simulink model "electricUAV"  (R2019a)
settings: Solver=VariableStepAuto  StartTime=0.0  StopTime=10.0  RelTol=1e-3
model workspace (MAT data in the model file):
  Var = 0
  architecture_gsCommands = Simulink.Bus
  architecture_gsCommands.Alignment = -1
  architecture_gsCommands.Elements_internal(1) = Simulink.BusElement
  architecture_gsCommands.Elements_internal(1).DimensionsMode = 'Fixed'
  architecture_gsCommands.Elements_internal(1).SamplingMode = 'Sample based'
  architecture_gsCommands.Elements_internal(1).SampleTime = -1
  architecture_gsCommands.Elements_internal(1).Name = 'apConfigParams'
  architecture_gsCommands.Elements_internal(1).DataType_internal = 'Bus: param_value_bus'
  architecture_gsCommands.Elements_internal(1).Complexity = 'real'
  architecture_gsCommands.Elements_internal(1).Dimensions = 1
  architecture_gsCommands.Elements_internal(2) = Simulink.BusElement
  architecture_gsCommands.Elements_internal(2).DimensionsMode = 'Fixed'
  architecture_gsCommands.Elements_internal(2).SamplingMode = 'Sample based'
  architecture_gsCommands.Elements_internal(2).SampleTime = -1
  architecture_gsCommands.Elements_internal(2).Name = 'gsCommands'
  architecture_gsCommands.Elements_internal(2).DataType_internal = 'Bus: gs_commands_bus'
  architecture_gsCommands.Elements_internal(2).Complexity = 'real'
  architecture_gsCommands.Elements_internal(2).Dimensions = 1
  architecture_gsCommands.Elements_internal(3) = Simulink.BusElement
  architecture_gsCommands.Elements_internal(3).DimensionsMode = 'Fixed'
  architecture_gsCommands.Elements_internal(3).SamplingMode = 'Sample based'
  architecture_gsCommands.Elements_internal(3).SampleTime = -1
  architecture_gsCommands.Elements_internal(3).Name = 'uavMission'
  architecture_gsCommands.Elements_internal(3).DataType_internal = 'Bus: mission_item_bus'
  architecture_gsCommands.Elements_internal(3).Complexity = 'real'
  architecture_gsCommands.Elements_internal(3).Dimensions = 1
  architecture_gsCommands.DataScope = 'Auto'
  ctrlSrfcDeflection = Simulink.Bus
  ctrlSrfcDeflection.Alignment = -1
  ctrlSrfcDeflection.Elements_internal(1) = Simulink.BusElement
  ctrlSrfcDeflection.Elements_internal(1).DimensionsMode = 'Fixed'
  ctrlSrfcDeflection.Elements_internal(1).SamplingMode = 'Sample based'
  ctrlSrfcDeflection.Elements_internal(1).SampleTime = -1
  ctrlSrfcDeflection.Elements_internal(1).Name = 'dA_dF'
  ctrlSrfcDeflection.Elements_internal(1).DataType_internal = 'double'
  ctrlSrfcDeflection.Elements_internal(1).Complexity = 'real'
  ctrlSrfcDeflection.Elements_internal(1).Dimensions = 1
  ctrlSrfcDeflection.Elements_internal(2) = Simulink.BusElement
  ctrlSrfcDeflection.Elements_internal(2).DimensionsMode = 'Fixed'
  ctrlSrfcDeflection.Elements_internal(2).SamplingMode = 'Sample based'
  ctrlSrfcDeflection.Elements_internal(2).SampleTime = -1
  ctrlSrfcDeflection.Elements_internal(2).Name = 'dT'
  ctrlSrfcDeflection.Elements_internal(2).DataType_internal = 'double'
  ctrlSrfcDeflection.Elements_internal(2).Complexity = 'real'
  ctrlSrfcDeflection.Elements_internal(2).Dimensions = 1
  ctrlSrfcDeflection.Elements_internal(3) = Simulink.BusElement
  ctrlSrfcDeflection.Elements_internal(3).DimensionsMode = 'Fixed'
  ctrlSrfcDeflection.Elements_internal(3).SamplingMode = 'Sample based'
  ctrlSrfcDeflection.Elements_internal(3).SampleTime = -1
  ctrlSrfcDeflection.Elements_internal(3).Name = 'dR_dE'
  ctrlSrfcDeflection.Elements_internal(3).DataType_internal = 'double'
  ctrlSrfcDeflection.Elements_internal(3).Complexity = 'real'
  ctrlSrfcDeflection.Elements_internal(3).Dimensions = 1
  ctrlSrfcDeflection.DataScope = 'Auto'
  gs_commands_bus = Simulink.Bus
  gs_commands_bus.Alignment = -1
  gs_commands_bus.Elements_internal(1) = Simulink.BusElement
  gs_commands_bus.Elements_internal(1).DimensionsMode = 'Fixed'
  gs_commands_bus.Elements_internal(1).SamplingMode = 'Sample based'
  gs_commands_bus.Elements_internal(1).SampleTime = -1
  gs_commands_bus.Elements_internal(1).Description = 'Return to Base Command'
  gs_commands_bus.Elements_internal(1).Name = 'RTB'
  gs_commands_bus.Elements_internal(1).DataType_internal = 'uint8'
  gs_commands_bus.Elements_internal(1).Complexity = 'real'
  gs_commands_bus.Elements_internal(1).Dimensions = 1
  gs_commands_bus.Elements_internal(2) = Simulink.BusElement
  gs_commands_bus.Elements_internal(2).DimensionsMode = 'Fixed'
  gs_commands_bus.Elements_internal(2).SamplingMode = 'Sample based'
  gs_commands_bus.Elements_internal(2).SampleTime = -1
  gs_commands_bus.Elements_internal(2).Description = 'Airspeed Commanded by the GS'
  gs_commands_bus.Elements_internal(2).Name = 'U_c'
  gs_commands_bus.Elements_internal(2).DataType_internal = 'single'
  gs_commands_bus.Elements_internal(2).Complexity = 'real'
  gs_commands_bus.Elements_internal(2).Dimensions = 1
  gs_commands_bus.Elements_internal(3) = Simulink.BusElement
  gs_commands_bus.Elements_internal(3).DimensionsMode = 'Fixed'
  gs_commands_bus.Elements_internal(3).SamplingMode = 'Sample based'
  gs_commands_bus.Elements_internal(3).SampleTime = -1
  gs_commands_bus.Elements_internal(3).Description = 'Turnrate command when in mid Level Commands guidance mode'
  gs_commands_bus.Elements_internal(3).Name = 'psiDot_c_mdiLevel'
  gs_commands_bus.Elements_internal(3).DataType_internal = 'single'
  gs_commands_bus.Elements_internal(3).Complexity = 'real'
  gs_commands_bus.Elements_internal(3).Dimensions = 1
  gs_commands_bus.Elements_internal(4) = Simulink.BusElement
  gs_commands_bus.Elements_internal(4).DimensionsMode = 'Fixed'
  gs_commands_bus.Elements_internal(4).SamplingMode = 'Sample based'
  gs_commands_bus.Elements_internal(4).SampleTime = -1
  gs_commands_bus.Elements_internal(4).Description = 'Commanded altitude when in Mid Level Commands Mode. Also used as the altitude for RTB'
  gs_commands_bus.Elements_internal(4).Name = 'h_c_midLevel'
  gs_commands_bus.Elements_internal(4).DataType_internal = 'single'
  gs_commands_bus.Elements_internal(4).Complexity = 'real'
  gs_commands_bus.Elements_internal(4).Dimensions = 1
  gs_commands_bus.Elements_internal(5) = Simulink.BusElement
  gs_commands_bus.Elements_internal(5).DimensionsMode = 'Fixed'
  gs_commands_bus.Elements_internal(5).SamplingMode = 'Sample based'
  gs_commands_bus.Elements_internal(5).SampleTime = -1
  gs_commands_bus.Elements_internal(5).Name = 'isManualModeOn'
  gs_commands_bus.Elements_internal(5).DataType_internal = 'uint8'
  gs_commands_bus.Elements_internal(5).Complexity = 'real'
  gs_commands_bus.Elements_internal(5).Dimensions = 1
  gs_commands_bus.Elements_internal(6) = Simulink.BusElement
  gs_commands_bus.Elements_internal(6).DimensionsMode = 'Fixed'
  gs_commands_bus.Elements_internal(6).SamplingMode = 'Sample based'
  gs_commands_bus.Elements_internal(6).SampleTime = -1
  gs_commands_bus.Elements_internal(6).Name = 'viewPointIdx'
  gs_commands_bus.Elements_internal(6).DataType_internal = 'uint8'
  gs_commands_bus.Elements_internal(6).Complexity = 'real'
  gs_commands_bus.Elements_internal(6).Dimensions = 1
  gs_commands_bus.Elements_internal(7) = Simulink.BusElement
  gs_commands_bus.Elements_internal(7).DimensionsMode = 'Fixed'
  gs_commands_bus.Elements_internal(7).SamplingMode = 'Sample based'
  gs_commands_bus.Elements_internal(7).SampleTime = -1
  gs_commands_bus.Elements_internal(7).Name = 'guidanceMode'
  gs_commands_bus.Elements_internal(7).DataType_internal = 'uint8'
  gs_commands_bus.Elements_internal(7).Complexity = 'real'
  gs_commands_bus.Elements_internal(7).Dimensions = 1
  gs_commands_bus.DataScope = 'Auto'
  lightCmds = Simulink.Bus
  lightCmds.Alignment = -1
  lightCmds.Elements_internal(1) = Simulink.BusElement
  lightCmds.Elements_internal(1).DimensionsMode = 'Fixed'
  lightCmds.Elements_internal(1).SamplingMode = 'Sample based'
  lightCmds.Elements_internal(1).SampleTime = -1
  lightCmds.Elements_internal(1).Name = 'NavigationLights'
  lightCmds.Elements_internal(1).DataType_internal = 'double'
  lightCmds.Elements_internal(1).Complexity = 'real'
  lightCmds.Elements_internal(1).Dimensions = 1
  lightCmds.Elements_internal(2) = Simulink.BusElement
  lightCmds.Elements_internal(2).DimensionsMode = 'Fixed'
  lightCmds.Elements_internal(2).SamplingMode = 'Sample based'
  lightCmds.Elements_internal(2).SampleTime = -1
  lightCmds.Elements_internal(2).Name = 'LandingStrobe'
  lightCmds.Elements_internal(2).DataType_internal = 'double'
  lightCmds.Elements_internal(2).Complexity = 'real'
  lightCmds.Elements_internal(2).Dimensions = 1
  lightCmds.DataScope = 'Auto'
  mission_item_bus = Simulink.Bus
  mission_item_bus.Alignment = -1
  mission_item_bus.Elements_internal(1) = Simulink.BusElement
  mission_item_bus.Elements_internal(1).DimensionsMode = 'Fixed'
  mission_item_bus.Elements_internal(1).SamplingMode = 'Sample based'
  mission_item_bus.Elements_internal(1).SampleTime = -1
  mission_item_bus.Elements_internal(1).Description = 'PARAM1, see MAV_CMD enum'
  mission_item_bus.Elements_internal(1).Name = 'param1'
  mission_item_bus.Elements_internal(1).DataType_internal = 'single'
  mission_item_bus.Elements_internal(1).Complexity = 'real'
  mission_item_bus.Elements_internal(1).Dimensions = 1
  mission_item_bus.Elements_internal(2) = Simulink.BusElement
  mission_item_bus.Elements_internal(2).DimensionsMode = 'Fixed'
  mission_item_bus.Elements_internal(2).SamplingMode = 'Sample based'
  mission_item_bus.Elements_internal(2).SampleTime = -1
  mission_item_bus.Elements_internal(2).Description = 'PARAM4, see MAV_CMD enum'
  mission_item_bus.Elements_internal(2).Name = 'param4'
  mission_item_bus.Elements_internal(2).DataType_internal = 'single'
  mission_item_bus.Elements_internal(2).Complexity = 'real'
  mission_item_bus.Elements_internal(2).Dimensions = 1
  mission_item_bus.Elements_internal(3) = Simulink.BusElement
  mission_item_bus.Elements_internal(3).DimensionsMode = 'Fixed'
  mission_item_bus.Elements_internal(3).SamplingMode = 'Sample based'
  mission_item_bus.Elements_internal(3).SampleTime = -1
  mission_item_bus.Elements_internal(3).Description = 'PARAM3, see MAV_CMD enum'
  mission_item_bus.Elements_internal(3).Name = 'param3'
  mission_item_bus.Elements_internal(3).DataType_internal = 'single'
  mission_item_bus.Elements_internal(3).Complexity = 'real'
  mission_item_bus.Elements_internal(3).Dimensions = 1
  mission_item_bus.Elements_internal(4) = Simulink.BusElement
  mission_item_bus.Elements_internal(4).DimensionsMode = 'Fixed'
  mission_item_bus.Elements_internal(4).SamplingMode = 'Sample based'
  mission_item_bus.Elements_internal(4).SampleTime = -1
  mission_item_bus.Elements_internal(4).Description = 'false:0, true:1'
  mission_item_bus.Elements_internal(4).Name = 'current'
  mission_item_bus.Elements_internal(4).DataType_internal = 'uint8'
  mission_item_bus.Elements_internal(4).Complexity = 'real'
  mission_item_bus.Elements_internal(4).Dimensions = 1
  mission_item_bus.Elements_internal(5) = Simulink.BusElement
  mission_item_bus.Elements_internal(5).DimensionsMode = 'Fixed'
  mission_item_bus.Elements_internal(5).SamplingMode = 'Sample based'
  mission_item_bus.Elements_internal(5).SampleTime = -1
  mission_item_bus.Elements_internal(5).Description = 'PARAM2, see MAV_CMD enum'
  mission_item_bus.Elements_internal(5).Name = 'param2'
  mission_item_bus.Elements_internal(5).DataType_internal = 'single'
  mission_item_bus.Elements_internal(5).Complexity = 'real'
  mission_item_bus.Elements_internal(5).Dimensions = 1
  mission_item_bus.Elements_internal(6) = Simulink.BusElement
  mission_item_bus.Elements_internal(6).DimensionsMode = 'Fixed'
  mission_item_bus.Elements_internal(6).SamplingMode = 'Sample based'
  mission_item_bus.Elements_internal(6).SampleTime = -1
  mission_item_bus.Elements_internal(6).Description = 'PARAM5 / local: x position, global: latitude'
  mission_item_bus.Elements_internal(6).Name = 'x'
  mission_item_bus.Elements_internal(6).DataType_internal = 'single'
  mission_item_bus.Elements_internal(6).Complexity = 'real'
  mission_item_bus.Elements_internal(6).Dimensions = 1
  mission_item_bus.Elements_internal(7) = Simulink.BusElement
  mission_item_bus.Elements_internal(7).DimensionsMode = 'Fixed'
  mission_item_bus.Elements_internal(7).SamplingMode = 'Sample based'
  mission_item_bus.Elements_internal(7).SampleTime = -1
  mission_item_bus.Elements_internal(7).Description = 'PARAM6 / y position: global: longitude'
  mission_item_bus.Elements_internal(7).Name = 'y'
  mission_item_bus.Elements_internal(7).DataType_internal = 'single'
  mission_item_bus.Elements_internal(7).Complexity = 'real'
  mission_item_bus.Elements_internal(7).Dimensions = 1
  mission_item_bus.Elements_internal(8) = Simulink.BusElement
  mission_item_bus.Elements_internal(8).DimensionsMode = 'Fixed'
  mission_item_bus.Elements_internal(8).SamplingMode = 'Sample based'
  mission_item_bus.Elements_internal(8).SampleTime = -1
  mission_item_bus.Elements_internal(8).Description = 'The scheduled action for the waypoint. see MAV_CMD in common.xml MAVLink specs'
  mission_item_bus.Elements_internal(8).Name = 'command'
  mission_item_bus.Elements_internal(8).DataType_internal = 'uint16'
  mission_item_bus.Elements_internal(8).Complexity = 'real'
  mission_item_bus.Elements_internal(8).Dimensions = 1
  mission_item_bus.Elements_internal(9) = Simulink.BusElement
  mission_item_bus.Elements_internal(9).DimensionsMode = 'Fixed'
  mission_item_bus.Elements_internal(9).SamplingMode = 'Sample based'
  mission_item_bus.Elements_internal(9).SampleTime = -1
  mission_item_bus.Elements_internal(9).Description = 'PARAM7 / z position: global: altitude (relative or absolute, depending on frame.'
  mission_item_bus.Elements_internal(9).Name = 'z'
  mission_item_bus.Elements_internal(9).DataType_internal = 'single'
  mission_item_bus.Elements_internal(9).Complexity = 'real'
  mission_item_bus.Elements_internal(9).Dimensions = 1
  mission_item_bus.Elements_internal(10) = Simulink.BusElement
  mission_item_bus.Elements_internal(10).DimensionsMode = 'Fixed'
  mission_item_bus.Elements_internal(10).SamplingMode = 'Sample based'
  mission_item_bus.Elements_internal(10).SampleTime = -1
  mission_item_bus.Elements_internal(10).Description = 'System ID'
  mission_item_bus.Elements_internal(10).Name = 'target_system'
  mission_item_bus.Elements_internal(10).DataType_internal = 'uint8'
  mission_item_bus.Elements_internal(10).Complexity = 'real'
  mission_item_bus.Elements_internal(10).Dimensions = 1
  mission_item_bus.Elements_internal(11) = Simulink.BusElement
  mission_item_bus.Elements_internal(11).DimensionsMode = 'Fixed'
  mission_item_bus.Elements_internal(11).SamplingMode = 'Sample based'
  mission_item_bus.Elements_internal(11).SampleTime = -1
  mission_item_bus.Elements_internal(11).Description = 'Sequence'
  mission_item_bus.Elements_internal(11).Name = 'seq'
  mission_item_bus.Elements_internal(11).DataType_internal = 'uint16'
  mission_item_bus.Elements_internal(11).Complexity = 'real'
  mission_item_bus.Elements_internal(11).Dimensions = 1
  mission_item_bus.Elements_internal(12) = Simulink.BusElement
  mission_item_bus.Elements_internal(12).DimensionsMode = 'Fixed'
  mission_item_bus.Elements_internal(12).SamplingMode = 'Sample based'
  mission_item_bus.Elements_internal(12).SampleTime = -1
  mission_item_bus.Elements_internal(12).Description = 'Mission type, see MAV_MISSION_TYPE'
  mission_item_bus.Elements_internal(12).Name = 'mission_type'
  mission_item_bus.Elements_internal(12).DataType_internal = 'uint8'
  mission_item_bus.Elements_internal(12).Complexity = 'real'
  mission_item_bus.Elements_internal(12).Dimensions = 1
  mission_item_bus.Elements_internal(13) = Simulink.BusElement
  mission_item_bus.Elements_internal(13).DimensionsMode = 'Fixed'
  mission_item_bus.Elements_internal(13).SamplingMode = 'Sample based'
  mission_item_bus.Elements_internal(13).SampleTime = -1
  mission_item_bus.Elements_internal(13).Description = 'The coordinate system of the waypoint. see MAV_FRAME in mavlink_types.h'
  mission_item_bus.Elements_internal(13).Name = 'frame'
  mission_item_bus.Elements_internal(13).DataType_internal = 'uint8'
  mission_item_bus.Elements_internal(13).Complexity = 'real'
  mission_item_bus.Elements_internal(13).Dimensions = 1
  mission_item_bus.Elements_internal(14) = Simulink.BusElement
  mission_item_bus.Elements_internal(14).DimensionsMode = 'Fixed'
  mission_item_bus.Elements_internal(14).SamplingMode = 'Sample based'
  mission_item_bus.Elements_internal(14).SampleTime = -1
  mission_item_bus.Elements_internal(14).Description = 'Component ID'
  mission_item_bus.Elements_internal(14).Name = 'target_component'
  mission_item_bus.Elements_internal(14).DataType_internal = 'uint8'
  mission_item_bus.Elements_internal(14).Complexity = 'real'
  mission_item_bus.Elements_internal(14).Dimensions = 1
  mission_item_bus.Elements_internal(15) = Simulink.BusElement
  mission_item_bus.Elements_internal(15).DimensionsMode = 'Fixed'
  mission_item_bus.Elements_internal(15).SamplingMode = 'Sample based'
  mission_item_bus.Elements_internal(15).SampleTime = -1
  mission_item_bus.Elements_internal(15).Description = 'autocontinue to next wp'
  mission_item_bus.Elements_internal(15).Name = 'autocontinue'
  mission_item_bus.Elements_internal(15).DataType_internal = 'uint8'
  mission_item_bus.Elements_internal(15).Complexity = 'real'
  mission_item_bus.Elements_internal(15).Dimensions = 1
  mission_item_bus.DataScope = 'Auto'
  operatorCmds = Simulink.Bus
  operatorCmds.Alignment = -1
  operatorCmds.Elements_internal(1) = Simulink.BusElement
  operatorCmds.Elements_internal(1).DimensionsMode = 'Fixed'
  operatorCmds.Elements_internal(1).SamplingMode = 'Sample based'
  operatorCmds.Elements_internal(1).SampleTime = -1
  operatorCmds.Elements_internal(1).Name = 'RetractorCmds'
  operatorCmds.Elements_internal(1).DataType_internal = 'double'
  operatorCmds.Elements_internal(1).Complexity = 'real'
  operatorCmds.Elements_internal(1).Dimensions = 1
  operatorCmds.Elements_internal(2) = Simulink.BusElement
  operatorCmds.Elements_internal(2).DimensionsMode = 'Fixed'
  operatorCmds.Elements_internal(2).SamplingMode = 'Sample based'
  operatorCmds.Elements_internal(2).SampleTime = -1
  operatorCmds.Elements_internal(2).Name = 'PTZCmds'
  operatorCmds.Elements_internal(2).DataType_internal = 'double'
  operatorCmds.Elements_internal(2).Complexity = 'real'
  operatorCmds.Elements_internal(2).Dimensions = 1
  operatorCmds.DataScope = 'Auto'
  param_value_bus = Simulink.Bus
  param_value_bus.Alignment = -1
  param_value_bus.Elements_internal(1) = Simulink.BusElement
  param_value_bus.Elements_internal(1).DimensionsMode = 'Fixed'
  param_value_bus.Elements_internal(1).SamplingMode = 'Sample based'
  param_value_bus.Elements_internal(1).SampleTime = -1
  param_value_bus.Elements_internal(1).Description = 'Onboard parameter value'
  param_value_bus.Elements_internal(1).Name = 'param_value'
  param_value_bus.Elements_internal(1).DataType_internal = 'single'
  param_value_bus.Elements_internal(1).Complexity = 'real'
  param_value_bus.Elements_internal(1).Dimensions = 1
  param_value_bus.Elements_internal(2) = Simulink.BusElement
  param_value_bus.Elements_internal(2).DimensionsMode = 'Fixed'
  param_value_bus.Elements_internal(2).SamplingMode = 'Sample based'
  param_value_bus.Elements_internal(2).SampleTime = -1
  param_value_bus.Elements_internal(2).Description = 'Index of this onboard parameter'
  param_value_bus.Elements_internal(2).Name = 'param_index'
  param_value_bus.Elements_internal(2).DataType_internal = 'uint16'
  param_value_bus.Elements_internal(2).Complexity = 'real'
  param_value_bus.Elements_internal(2).Dimensions = 1
  param_value_bus.Elements_internal(3) = Simulink.BusElement
  param_value_bus.Elements_internal(3).DimensionsMode = 'Fixed'
  param_value_bus.Elements_internal(3).SamplingMode = 'Sample based'
  param_value_bus.Elements_internal(3).SampleTime = -1
  param_value_bus.Elements_internal(3).Description = 'Total number of onboard parameters'
  param_value_bus.Elements_internal(3).Name = 'param_count'
  param_value_bus.Elements_internal(3).DataType_internal = 'uint16'
  param_value_bus.Elements_internal(3).Complexity = 'real'
  param_value_bus.Elements_internal(3).Dimensions = 1
  param_value_bus.Elements_internal(4) = Simulink.BusElement
  param_value_bus.Elements_internal(4).DimensionsMode = 'Fixed'
  param_value_bus.Elements_internal(4).SamplingMode = 'Sample based'
  param_value_bus.Elements_internal(4).SampleTime = -1
  param_value_bus.Elements_internal(4).Description = 'Onboard parameter id, terminated by NULL if the length is less than 16 human-readable chars and WITHOUT null termination (NULL) byte if the length is exactly 16 chars - applications have to provide 16+1 bytes storage if the ID is stored as string'
  param_value_bus.Elements_internal(4).Name = 'param_id'
  param_value_bus.Elements_internal(4).DataType_internal = 'int8'
  param_value_bus.Elements_internal(4).Complexity = 'real'
  param_value_bus.Elements_internal(4).Dimensions = 16
  param_value_bus.Elements_internal(5) = Simulink.BusElement
  param_value_bus.Elements_internal(5).DimensionsMode = 'Fixed'
  param_value_bus.Elements_internal(5).SamplingMode = 'Sample based'
  param_value_bus.Elements_internal(5).SampleTime = -1
  param_value_bus.Elements_internal(5).Description = 'Onboard parameter type: see the MAV_PARAM_TYPE enum for supported data types.'
  param_value_bus.Elements_internal(5).Name = 'param_type'
  param_value_bus.Elements_internal(5).DataType_internal = 'uint8'
  param_value_bus.Elements_internal(5).Complexity = 'real'
  param_value_bus.Elements_internal(5).Dimensions = 1
  param_value_bus.DataScope = 'Auto'
settings Model: OrderedModelArguments=off  Creator=pshukla  LastModifiedBy=lizarraga

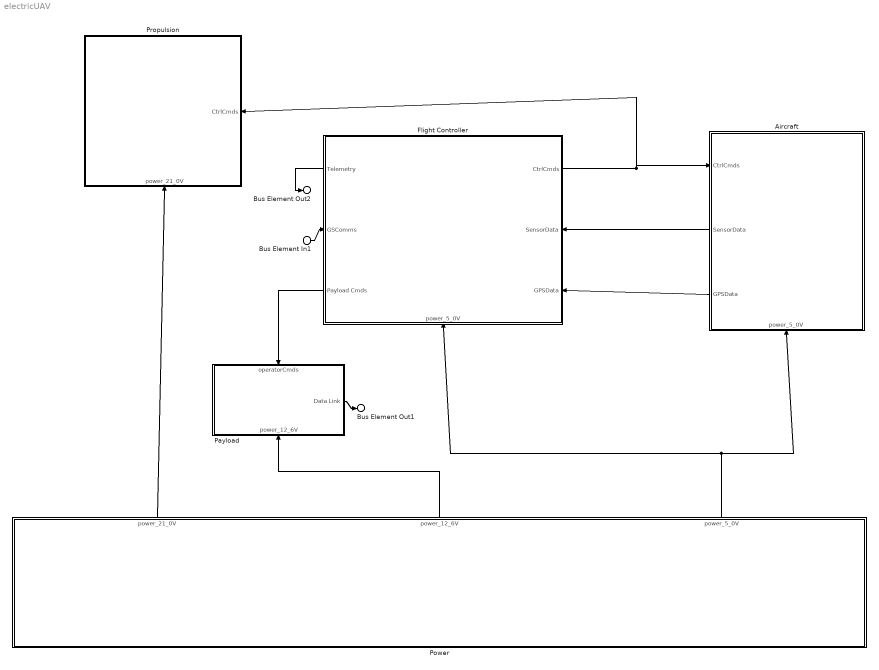
== system electricUAV ==
  Bus Element In1 : Inport  PortName=GS Communication
  Aircraft : Subsystem
      settings: PortSchema="{\"entries\":[{\"content\":{\"headerSize\":26,\"margin\":15,\"minimumSpacing\":25,\"sides\":[{\"content\":{\"connectorIds\":[\"In2\",\"Out1\",\"Out2\"]},\"type\":\"ConnectorPlacement.EquallySpacedRectSide\",\"uuid\":\"5864bfaa-27bf-4dc4-ac35-2a67754e9235\"},{\"content\":{\"connectorIds\":[],\"side\":\"RIGHT\"},\"type\":\"ConnectorPlacement.EquallySpacedRectSide\",\"uuid\":\"1b67a812-6201-4dd3-b7dd-96f38505ac3f\"},{\"content\":{\"connectorIds\":[],\"side\":\"TOP\"},\"type\":\"ConnectorPlacement.EquallySpacedRectSide\",\"uuid\":\"0ccb1f06-40bd-43a7-ae7f-56a6fcc507bd\"},{\"content\":{\"connectorIds\":[\"In1\"],\"side\":\"BOTTOM\"},\"type\":\"ConnectorPlacement.EquallySpacedRectSide\",\"uuid\":\"b85c3588-b067-49c6-8cfc-8b359955ba08\"}]},\"type\":\"ConnectorPlacement.EquallySpacedConnector\",\"uuid\":\"adb7d5a4-9c70-4105-bc6e-780ed1523c48\"}],\"packageUris\":[\"http:\\/\\/schema.mathworks.com\\/mf0\\/Connector\\/19700101\"],\"version\":\"1.0\"}"
  Flight Controller : Subsystem
      settings: PortSchema="{\"entries\":[{\"content\":{\"headerSize\":26,\"margin\":15,\"minimumSpacing\":25,\"sides\":[{\"content\":{\"connectorIds\":[\"Out3\",\"In4\",\"Out2\"]},\"type\":\"ConnectorPlacement.EquallySpacedRectSide\",\"uuid\":\"288187f8-f80a-4535-8eff-6998f4e932c0\"},{\"content\":{\"connectorIds\":[\"Out1\",\"In2\",\"In3\"],\"side\":\"RIGHT\"},\"type\":\"ConnectorPlacement.EquallySpacedRectSide\",\"uuid\":\"d1e22774-cdd2-4e71-94b1-3e938d9d16f6\"},{\"content\":{\"connectorIds\":[],\"side\":\"TOP\"},\"type\":\"ConnectorPlacement.EquallySpacedRectSide\",\"uuid\":\"890411bd-a9cd-40b1-a683-0574f0cd14d7\"},{\"content\":{\"connectorIds\":[\"In1\"],\"side\":\"BOTTOM\"},\"type\":\"ConnectorPlacement.EquallySpacedRectSide\",\"uuid\":\"5b2b87a3-00cb-493f-9187-a9231b1dbd9e\"}]},\"type\":\"ConnectorPlacement.EquallySpacedConnector\",\"uuid\":\"f677e6f7-ddb0-43ad-ab3a-7892dac74d79\"}],\"packageUris\":[\"http:\\/\\/schema.mathworks.com\\/mf0\\/Connector\\/19700101\"],\"version\":\"1.0\"}"
  Payload : Subsystem
      settings: PortSchema="{\"entries\":[{\"content\":{\"headerSize\":26,\"margin\":15,\"minimumSpacing\":25,\"sides\":[{\"content\":{\"connectorIds\":[]},\"type\":\"ConnectorPlacement.EquallySpacedRectSide\",\"uuid\":\"288187f8-f80a-4535-8eff-6998f4e932c0\"},{\"content\":{\"connectorIds\":[\"Out1\"],\"side\":\"RIGHT\"},\"type\":\"ConnectorPlacement.EquallySpacedRectSide\",\"uuid\":\"d1e22774-cdd2-4e71-94b1-3e938d9d16f6\"},{\"content\":{\"connectorIds\":[\"In2\"],\"side\":\"TOP\"},\"type\":\"ConnectorPlacement.EquallySpacedRectSide\",\"uuid\":\"890411bd-a9cd-40b1-a683-0574f0cd14d7\"},{\"content\":{\"connectorIds\":[\"In1\"],\"side\":\"BOTTOM\"},\"type\":\"ConnectorPlacement.EquallySpacedRectSide\",\"uuid\":\"ac2f29b9-61c6-4e35-85f4-3f1356623504\"}]},\"type\":\"ConnectorPlacement.EquallySpacedConnector\",\"uuid\":\"f677e6f7-ddb0-43ad-ab3a-7892dac74d79\"}],\"packageUris\":[\"http:\\/\\/schema.mathworks.com\\/mf0\\/Connector\\/19700101\"],\"version\":\"1.0\"}"
  Power : Subsystem
      settings: PortSchema="{\"entries\":[{\"content\":{\"headerSize\":26,\"margin\":15,\"minimumSpacing\":25,\"sides\":[{\"content\":{\"connectorIds\":[]},\"type\":\"ConnectorPlacement.EquallySpacedRectSide\",\"uuid\":\"76636d8c-2a71-4cfe-9798-180c72f47694\"},{\"content\":{\"connectorIds\":[],\"side\":\"RIGHT\"},\"type\":\"ConnectorPlacement.EquallySpacedRectSide\",\"uuid\":\"872f7c71-0239-4d56-8641-47d463e7d626\"},{\"content\":{\"connectorIds\":[\"Out3\",\"Out2\",\"Out1\"],\"side\":\"TOP\"},\"type\":\"ConnectorPlacement.EquallySpacedRectSide\",\"uuid\":\"1d792a1c-d9fe-46f0-a4cc-898d179764e8\"}]},\"type\":\"ConnectorPlacement.EquallySpacedConnector\",\"uuid\":\"a92a26c6-31c1-4459-9e74-ec0692bdfd16\"}],\"packageUris\":[\"http:\\/\\/schema.mathworks.com\\/mf0\\/Connector\\/19700101\"],\"version\":\"1.0\"}"
  Propulsion : Subsystem
      settings: PortSchema="{\"entries\":[{\"content\":{\"headerSize\":26,\"margin\":15,\"minimumSpacing\":25,\"sides\":[{\"content\":{\"connectorIds\":[]},\"type\":\"ConnectorPlacement.EquallySpacedRectSide\",\"uuid\":\"288187f8-f80a-4535-8eff-6998f4e932c0\"},{\"content\":{\"connectorIds\":[\"In2\"],\"side\":\"RIGHT\"},\"type\":\"ConnectorPlacement.EquallySpacedRectSide\",\"uuid\":\"d1e22774-cdd2-4e71-94b1-3e938d9d16f6\"},{\"content\":{\"connectorIds\":[],\"side\":\"TOP\"},\"type\":\"ConnectorPlacement.EquallySpacedRectSide\",\"uuid\":\"890411bd-a9cd-40b1-a683-0574f0cd14d7\"},{\"content\":{\"connectorIds\":[\"In1\"],\"side\":\"BOTTOM\"},\"type\":\"ConnectorPlacement.EquallySpacedRectSide\",\"uuid\":\"d166b9ee-3d3a-4bd4-a932-7454a321b638\"}]},\"type\":\"ConnectorPlacement.EquallySpacedConnector\",\"uuid\":\"f677e6f7-ddb0-43ad-ab3a-7892dac74d79\"}],\"packageUris\":[\"http:\\/\\/schema.mathworks.com\\/mf0\\/Connector\\/19700101\"],\"version\":\"1.0\"}"
  Bus Element Out1 : Outport  PortName=Data Link
  Bus Element Out2 : Outport  Port=2  PortName=Telemetry
  wires:
  Payload/1(Data Link) -> Bus Element Out1/1
  Flight Controller/3(Telemetry) -> Bus Element Out2/1
  Flight Controller/2(Payload Cmds) -> Payload/2(operatorCmds)
  Power/3(power_21_0V) -> Propulsion/1(power_21_0V)
  Power/2(power_12_6V) -> Payload/1(power_12_6V)
  Bus Element In1/1 -> Flight Controller/4(GSComms)
  Flight Controller/1(CtrlCmds) -> Propulsion/2(CtrlCmds), Aircraft/2(CtrlCmds)
  Power/1(power_5_0V) -> Aircraft/1(power_5_0V), Flight Controller/1(power_5_0V)
  Aircraft/1(SensorData) -> Flight Controller/2(SensorData)
  Aircraft/2(GPSData) -> Flight Controller/3(GPSData)

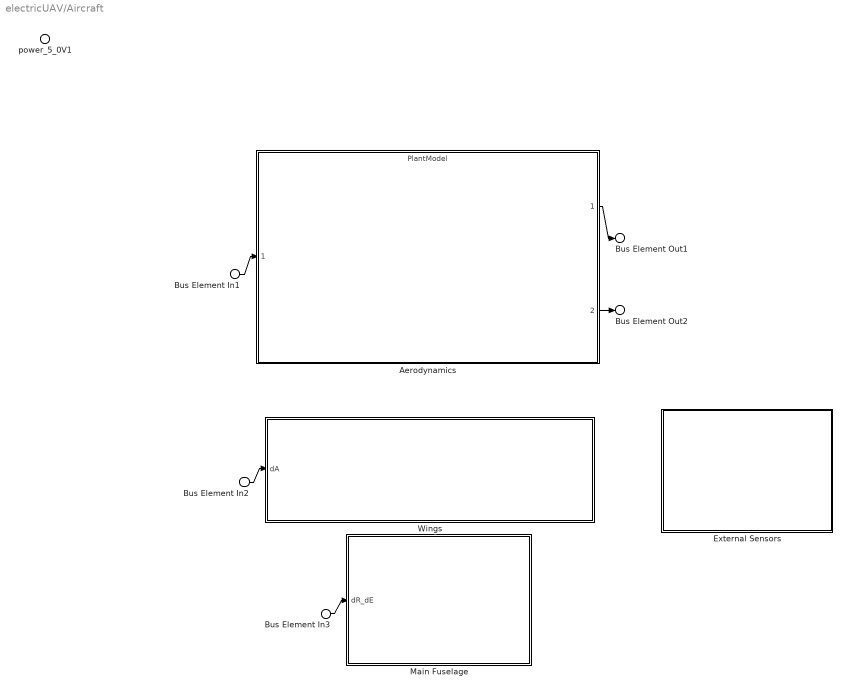
== system electricUAV/Aircraft ==
  power_5_0V1 : Inport  PortName=power_5_0V
  Bus Element In1 : Inport  Port=2  PortName=CtrlCmds
  Bus Element In2 : Inport  Port=2  PortName=CtrlCmds  Element=dA
  Bus Element In3 : Inport  Port=2  PortName=CtrlCmds  Element=dE_dE
  Aerodynamics : ModelReference  ModelNameDialog=PlantModel  SimulationMode=Normal  ModelReferenceVersion=1.375
      settings: PortSchema="{\"entries\":[{\"content\":{\"headerSize\":38,\"margin\":15,\"minimumSpacing\":25,\"sides\":[{\"content\":{\"connectorIds\":[\"In1\"]},\"type\":\"ConnectorPlacement.EquallySpacedRectSide\",\"uuid\":\"5864bfaa-27bf-4dc4-ac35-2a67754e9235\"},{\"content\":{\"connectorIds\":[\"Out1\",\"Out2\"],\"side\":\"RIGHT\"},\"type\":\"ConnectorPlacement.EquallySpacedRectSide\",\"uuid\":\"1b67a812-6201-4dd3-b7dd-96f38505ac3f\"},{\"content\":{\"connectorIds\":[],\"side\":\"TOP\"},\"type\":\"ConnectorPlacement.EquallySpacedRectSide\",\"uuid\":\"0ccb1f06-40bd-43a7-ae7f-56a6fcc507bd\"}]},\"type\":\"ConnectorPlacement.EquallySpacedConnector\",\"uuid\":\"adb7d5a4-9c70-4105-bc6e-780ed1523c48\"}],\"packageUris\":[\"http:\\/\\/schema.mathworks.com\\/mf0\\/Connector\\/19700101\"],\"version\":\"1.0\"}"
  External Sensors : Subsystem
      settings: PortSchema="{\"entries\":[{\"content\":{\"headerSize\":26,\"margin\":15,\"minimumSpacing\":25,\"sides\":[{\"content\":{\"connectorIds\":[]},\"type\":\"ConnectorPlacement.EquallySpacedRectSide\",\"uuid\":\"62bd5ee8-2365-4a2b-9d30-43e6a529a901\"},{\"content\":{\"connectorIds\":[],\"side\":\"RIGHT\"},\"type\":\"ConnectorPlacement.EquallySpacedRectSide\",\"uuid\":\"ad573e81-da6c-48c9-9164-7d3bad2ceb97\"},{\"content\":{\"connectorIds\":[],\"side\":\"TOP\"},\"type\":\"ConnectorPlacement.EquallySpacedRectSide\",\"uuid\":\"751ccae3-2e52-4144-859d-59b43885f9a5\"}]},\"type\":\"ConnectorPlacement.EquallySpacedConnector\",\"uuid\":\"5c6bf82f-fc67-4316-a7a6-96067f01ece3\"}],\"packageUris\":[\"http:\\/\\/schema.mathworks.com\\/mf0\\/Connector\\/19700101\"],\"version\":\"1.0\"}"
  Main Fuselage : Subsystem
      settings: PortSchema="{\"entries\":[{\"content\":{\"headerSize\":26,\"margin\":15,\"minimumSpacing\":25,\"sides\":[{\"content\":{\"connectorIds\":[\"In1\"]},\"type\":\"ConnectorPlacement.EquallySpacedRectSide\",\"uuid\":\"410c5b0f-08b5-48c1-aeab-ad32707f18cb\"},{\"content\":{\"connectorIds\":[],\"side\":\"RIGHT\"},\"type\":\"ConnectorPlacement.EquallySpacedRectSide\",\"uuid\":\"175f376c-06cb-43d8-93cf-cfe74288c6ca\"},{\"content\":{\"connectorIds\":[],\"side\":\"TOP\"},\"type\":\"ConnectorPlacement.EquallySpacedRectSide\",\"uuid\":\"49daa1ce-2b00-43ab-833d-e4aa679275fe\"}]},\"type\":\"ConnectorPlacement.EquallySpacedConnector\",\"uuid\":\"5fe6ec80-a25e-4dcf-8012-d525fb653d3d\"}],\"packageUris\":[\"http:\\/\\/schema.mathworks.com\\/mf0\\/Connector\\/19700101\"],\"version\":\"1.0\"}"
  Wings : Subsystem
      settings: PortSchema="{\"entries\":[{\"content\":{\"headerSize\":26,\"margin\":15,\"minimumSpacing\":25,\"sides\":[{\"content\":{\"connectorIds\":[\"In1\"]},\"type\":\"ConnectorPlacement.EquallySpacedRectSide\",\"uuid\":\"410c5b0f-08b5-48c1-aeab-ad32707f18cb\"},{\"content\":{\"connectorIds\":[],\"side\":\"RIGHT\"},\"type\":\"ConnectorPlacement.EquallySpacedRectSide\",\"uuid\":\"175f376c-06cb-43d8-93cf-cfe74288c6ca\"},{\"content\":{\"connectorIds\":[],\"side\":\"TOP\"},\"type\":\"ConnectorPlacement.EquallySpacedRectSide\",\"uuid\":\"49daa1ce-2b00-43ab-833d-e4aa679275fe\"}]},\"type\":\"ConnectorPlacement.EquallySpacedConnector\",\"uuid\":\"5fe6ec80-a25e-4dcf-8012-d525fb653d3d\"}],\"packageUris\":[\"http:\\/\\/schema.mathworks.com\\/mf0\\/Connector\\/19700101\"],\"version\":\"1.0\"}"
  Bus Element Out1 : Outport  PortName=SensorData
  Bus Element Out2 : Outport  Port=2  PortName=GPSData
  wires:
  Bus Element In2/1 -> Wings/1(dA)
  Bus Element In3/1 -> Main Fuselage/1(dR_dE)
  Bus Element In1/1 -> Aerodynamics/1
  Aerodynamics/1 -> Bus Element Out1/1
  Aerodynamics/2 -> Bus Element Out2/1

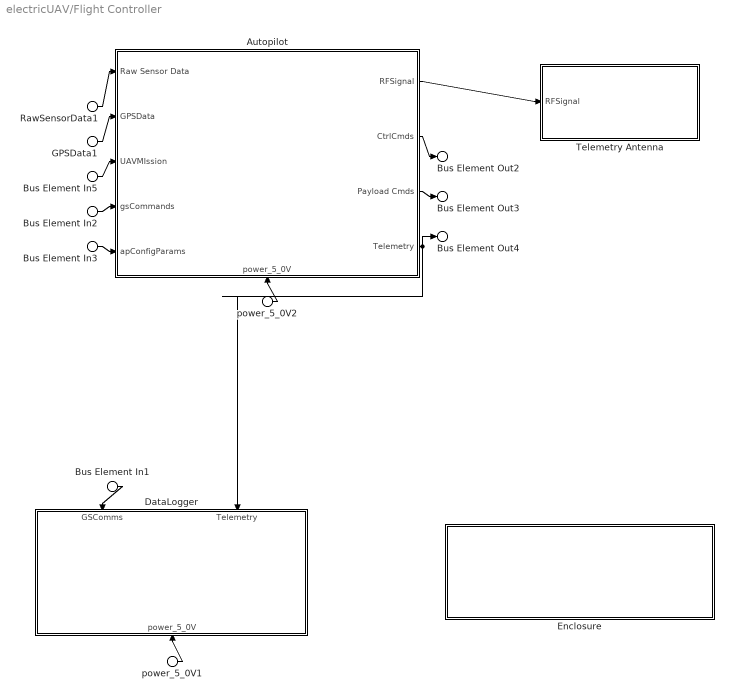
== system electricUAV/Flight Controller ==
  power_5_0V1 : Inport  PortName=power_5_0V
  power_5_0V2 : Inport  PortName=power_5_0V
  RawSensorData1 : Inport  Port=2  PortName=SensorData
  GPSData1 : Inport  Port=3  PortName=GPSData
  Bus Element In1 : Inport  Port=4  PortName=GSComms
  Bus Element In3 : Inport  Port=4  PortName=GSComms  Element=apConfigParams
  Bus Element In2 : Inport  Port=4  PortName=GSComms  Element=gsCommands
  Bus Element In5 : Inport  Port=4  PortName=GSComms  Element=uavMission
  Autopilot : Subsystem
      settings: PortSchema="{\"entries\":[{\"content\":{\"headerSize\":26,\"margin\":15,\"minimumSpacing\":25,\"sides\":[{\"content\":{\"connectorIds\":[\"In2\",\"In3\",\"In4\",\"In5\",\"In6\"]},\"type\":\"ConnectorPlacement.EquallySpacedRectSide\",\"uuid\":\"288187f8-f80a-4535-8eff-6998f4e932c0\"},{\"content\":{\"connectorIds\":[\"Out1\",\"Out2\",\"Out4\",\"Out3\"],\"side\":\"RIGHT\"},\"type\":\"ConnectorPlacement.EquallySpacedRectSide\",\"uuid\":\"d1e22774-cdd2-4e71-94b1-3e938d9d16f6\"},{\"content\":{\"connectorIds\":[],\"side\":\"TOP\"},\"type\":\"ConnectorPlacement.EquallySpacedRectSide\",\"uuid\":\"890411bd-a9cd-40b1-a683-0574f0cd14d7\"},{\"content\":{\"connectorIds\":[\"In1\"],\"side\":\"BOTTOM\"},\"type\":\"ConnectorPlacement.EquallySpacedRectSide\",\"uuid\":\"25c56d3a-a4ea-41c7-9d2f-6d234d9dfc35\"}]},\"type\":\"ConnectorPlacement.EquallySpacedConnector\",\"uuid\":\"f677e6f7-ddb0-43ad-ab3a-7892dac74d79\"}],\"packageUris\":[\"http:\\/\\/schema.mathworks.com\\/mf0\\/Connector\\/19700101\"],\"version\":\"1.0\"}"
  DataLogger : Subsystem
      settings: PortSchema="{\"entries\":[{\"content\":{\"headerSize\":26,\"margin\":15,\"minimumSpacing\":25,\"sides\":[{\"content\":{\"connectorIds\":[]},\"type\":\"ConnectorPlacement.EquallySpacedRectSide\",\"uuid\":\"410c5b0f-08b5-48c1-aeab-ad32707f18cb\"},{\"content\":{\"connectorIds\":[],\"side\":\"RIGHT\"},\"type\":\"ConnectorPlacement.EquallySpacedRectSide\",\"uuid\":\"175f376c-06cb-43d8-93cf-cfe74288c6ca\"},{\"content\":{\"connectorIds\":[\"In2\",\"In3\"],\"side\":\"TOP\"},\"type\":\"ConnectorPlacement.EquallySpacedRectSide\",\"uuid\":\"49daa1ce-2b00-43ab-833d-e4aa679275fe\"},{\"content\":{\"connectorIds\":[\"In1\"],\"side\":\"BOTTOM\"},\"type\":\"ConnectorPlacement.EquallySpacedRectSide\",\"uuid\":\"83f05929-3ae6-48a6-a28e-0b46043f22e2\"}]},\"type\":\"ConnectorPlacement.EquallySpacedConnector\",\"uuid\":\"5fe6ec80-a25e-4dcf-8012-d525fb653d3d\"}],\"packageUris\":[\"http:\\/\\/schema.mathworks.com\\/mf0\\/Connector\\/19700101\"],\"version\":\"1.0\"}"
  Enclosure : Subsystem
      settings: PortSchema="{\"entries\":[{\"content\":{\"headerSize\":26,\"margin\":15,\"minimumSpacing\":25,\"sides\":[{\"content\":{\"connectorIds\":[]},\"type\":\"ConnectorPlacement.EquallySpacedRectSide\",\"uuid\":\"1d3f3a23-636b-441d-85a6-b75e05b18389\"},{\"content\":{\"connectorIds\":[],\"side\":\"RIGHT\"},\"type\":\"ConnectorPlacement.EquallySpacedRectSide\",\"uuid\":\"e22d7e46-f58c-4c9d-8892-998381cd60e3\"},{\"content\":{\"connectorIds\":[],\"side\":\"TOP\"},\"type\":\"ConnectorPlacement.EquallySpacedRectSide\",\"uuid\":\"8b16ddbb-b471-4974-8372-55ce1efe9f0b\"}]},\"type\":\"ConnectorPlacement.EquallySpacedConnector\",\"uuid\":\"3aaecc83-0a24-4c0b-b096-52d61c24d002\"}],\"packageUris\":[\"http:\\/\\/schema.mathworks.com\\/mf0\\/Connector\\/19700101\"],\"version\":\"1.0\"}"
  Telemetry Antenna : Subsystem
      settings: PortSchema="{\"entries\":[{\"content\":{\"headerSize\":26,\"margin\":15,\"minimumSpacing\":25,\"sides\":[{\"content\":{\"connectorIds\":[\"In1\"]},\"type\":\"ConnectorPlacement.EquallySpacedRectSide\",\"uuid\":\"1d3f3a23-636b-441d-85a6-b75e05b18389\"},{\"content\":{\"connectorIds\":[],\"side\":\"RIGHT\"},\"type\":\"ConnectorPlacement.EquallySpacedRectSide\",\"uuid\":\"e22d7e46-f58c-4c9d-8892-998381cd60e3\"},{\"content\":{\"connectorIds\":[],\"side\":\"TOP\"},\"type\":\"ConnectorPlacement.EquallySpacedRectSide\",\"uuid\":\"8b16ddbb-b471-4974-8372-55ce1efe9f0b\"}]},\"type\":\"ConnectorPlacement.EquallySpacedConnector\",\"uuid\":\"3aaecc83-0a24-4c0b-b096-52d61c24d002\"}],\"packageUris\":[\"http:\\/\\/schema.mathworks.com\\/mf0\\/Connector\\/19700101\"],\"version\":\"1.0\"}"
  Bus Element Out2 : Outport  PortName=CtrlCmds
  Bus Element Out3 : Outport  Port=2  PortName=Payload Cmds
  Bus Element Out4 : Outport  Port=3  PortName=Telemetry
  wires:
  Autopilot/3(Telemetry) -> DataLogger/3(Telemetry), Bus Element Out4/1
  Bus Element In5/1 -> Autopilot/4(UAVMIssion)
  Autopilot/2(CtrlCmds) -> Bus Element Out2/1
  Autopilot/4(Payload Cmds) -> Bus Element Out3/1
  Autopilot/1(RFSignal) -> Telemetry Antenna/1(RFSignal)
  Bus Element In2/1 -> Autopilot/5(gsCommands)
  Bus Element In3/1 -> Autopilot/6(apConfigParams)
  GPSData1/1 -> Autopilot/3(GPSData)
  RawSensorData1/1 -> Autopilot/2(Raw Sensor Data)
  Bus Element In1/1 -> DataLogger/2(GSComms)
  power_5_0V1/1 -> DataLogger/1(power_5_0V)
  power_5_0V2/1 -> Autopilot/1(power_5_0V)

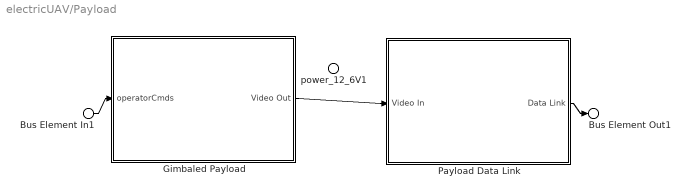
== system electricUAV/Payload ==
  power_12_6V1 : Inport  PortName=power_12_6V
  Bus Element In1 : Inport  Port=2  PortName=operatorCmds
  Gimbaled Payload : Subsystem
      settings: PortSchema="{\"entries\":[{\"content\":{\"headerSize\":26,\"margin\":15,\"minimumSpacing\":25,\"sides\":[{\"content\":{\"connectorIds\":[\"In1\"]},\"type\":\"ConnectorPlacement.EquallySpacedRectSide\",\"uuid\":\"288187f8-f80a-4535-8eff-6998f4e932c0\"},{\"content\":{\"connectorIds\":[\"Out1\"],\"side\":\"RIGHT\"},\"type\":\"ConnectorPlacement.EquallySpacedRectSide\",\"uuid\":\"d1e22774-cdd2-4e71-94b1-3e938d9d16f6\"},{\"content\":{\"connectorIds\":[],\"side\":\"TOP\"},\"type\":\"ConnectorPlacement.EquallySpacedRectSide\",\"uuid\":\"890411bd-a9cd-40b1-a683-0574f0cd14d7\"}]},\"type\":\"ConnectorPlacement.EquallySpacedConnector\",\"uuid\":\"f677e6f7-ddb0-43ad-ab3a-7892dac74d79\"}],\"packageUris\":[\"http:\\/\\/schema.mathworks.com\\/mf0\\/Connector\\/19700101\"],\"version\":\"1.0\"}"
  Payload Data Link : Subsystem
      settings: PortSchema="{\"entries\":[{\"content\":{\"headerSize\":26,\"margin\":15,\"minimumSpacing\":25,\"sides\":[{\"content\":{\"connectorIds\":[\"In1\"]},\"type\":\"ConnectorPlacement.EquallySpacedRectSide\",\"uuid\":\"288187f8-f80a-4535-8eff-6998f4e932c0\"},{\"content\":{\"connectorIds\":[\"Out1\"],\"side\":\"RIGHT\"},\"type\":\"ConnectorPlacement.EquallySpacedRectSide\",\"uuid\":\"d1e22774-cdd2-4e71-94b1-3e938d9d16f6\"},{\"content\":{\"connectorIds\":[],\"side\":\"TOP\"},\"type\":\"ConnectorPlacement.EquallySpacedRectSide\",\"uuid\":\"890411bd-a9cd-40b1-a683-0574f0cd14d7\"}]},\"type\":\"ConnectorPlacement.EquallySpacedConnector\",\"uuid\":\"f677e6f7-ddb0-43ad-ab3a-7892dac74d79\"}],\"packageUris\":[\"http:\\/\\/schema.mathworks.com\\/mf0\\/Connector\\/19700101\"],\"version\":\"1.0\"}"
  Bus Element Out1 : Outport  PortName=Data Link
  wires:
  Bus Element In1/1 -> Gimbaled Payload/1(operatorCmds)
  Gimbaled Payload/1(Video Out) -> Payload Data Link/1(Video In)
  Payload Data Link/1(Data Link) -> Bus Element Out1/1

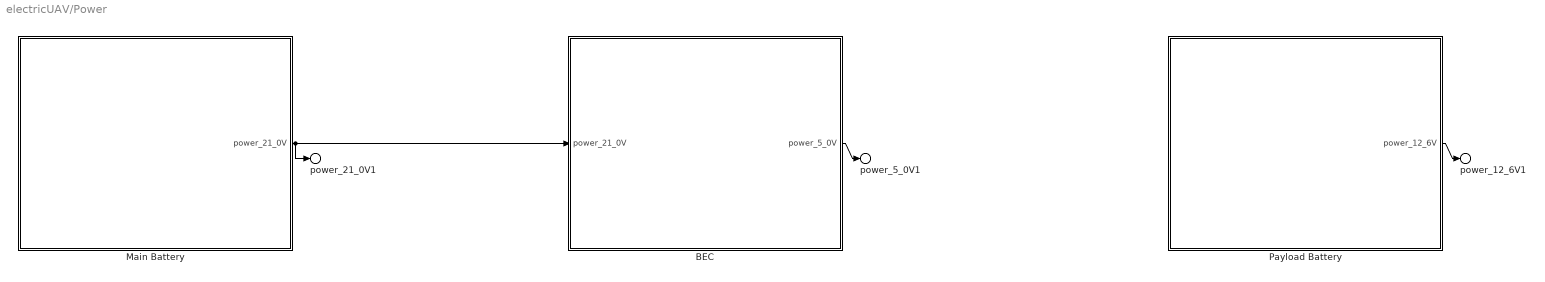
== system electricUAV/Power ==
  BEC : Subsystem
      settings: PortSchema="{\"entries\":[{\"content\":{\"headerSize\":26,\"margin\":15,\"minimumSpacing\":25,\"sides\":[{\"content\":{\"connectorIds\":[\"In1\"]},\"type\":\"ConnectorPlacement.EquallySpacedRectSide\",\"uuid\":\"76636d8c-2a71-4cfe-9798-180c72f47694\"},{\"content\":{\"connectorIds\":[\"Out1\"],\"side\":\"RIGHT\"},\"type\":\"ConnectorPlacement.EquallySpacedRectSide\",\"uuid\":\"872f7c71-0239-4d56-8641-47d463e7d626\"},{\"content\":{\"connectorIds\":[],\"side\":\"TOP\"},\"type\":\"ConnectorPlacement.EquallySpacedRectSide\",\"uuid\":\"1d792a1c-d9fe-46f0-a4cc-898d179764e8\"}]},\"type\":\"ConnectorPlacement.EquallySpacedConnector\",\"uuid\":\"a92a26c6-31c1-4459-9e74-ec0692bdfd16\"}],\"packageUris\":[\"http:\\/\\/schema.mathworks.com\\/mf0\\/Connector\\/19700101\"],\"version\":\"1.0\"}"
  Main Battery : Subsystem
      settings: PortSchema="{\"entries\":[{\"content\":{\"headerSize\":26,\"margin\":15,\"minimumSpacing\":25,\"sides\":[{\"content\":{\"connectorIds\":[]},\"type\":\"ConnectorPlacement.EquallySpacedRectSide\",\"uuid\":\"76636d8c-2a71-4cfe-9798-180c72f47694\"},{\"content\":{\"connectorIds\":[\"Out1\"],\"side\":\"RIGHT\"},\"type\":\"ConnectorPlacement.EquallySpacedRectSide\",\"uuid\":\"872f7c71-0239-4d56-8641-47d463e7d626\"},{\"content\":{\"connectorIds\":[],\"side\":\"TOP\"},\"type\":\"ConnectorPlacement.EquallySpacedRectSide\",\"uuid\":\"1d792a1c-d9fe-46f0-a4cc-898d179764e8\"}]},\"type\":\"ConnectorPlacement.EquallySpacedConnector\",\"uuid\":\"a92a26c6-31c1-4459-9e74-ec0692bdfd16\"}],\"packageUris\":[\"http:\\/\\/schema.mathworks.com\\/mf0\\/Connector\\/19700101\"],\"version\":\"1.0\"}"
  Payload Battery : Subsystem
      settings: PortSchema="{\"entries\":[{\"content\":{\"headerSize\":26,\"margin\":15,\"minimumSpacing\":25,\"sides\":[{\"content\":{\"connectorIds\":[]},\"type\":\"ConnectorPlacement.EquallySpacedRectSide\",\"uuid\":\"76636d8c-2a71-4cfe-9798-180c72f47694\"},{\"content\":{\"connectorIds\":[\"Out1\"],\"side\":\"RIGHT\"},\"type\":\"ConnectorPlacement.EquallySpacedRectSide\",\"uuid\":\"872f7c71-0239-4d56-8641-47d463e7d626\"},{\"content\":{\"connectorIds\":[],\"side\":\"TOP\"},\"type\":\"ConnectorPlacement.EquallySpacedRectSide\",\"uuid\":\"1d792a1c-d9fe-46f0-a4cc-898d179764e8\"}]},\"type\":\"ConnectorPlacement.EquallySpacedConnector\",\"uuid\":\"a92a26c6-31c1-4459-9e74-ec0692bdfd16\"}],\"packageUris\":[\"http:\\/\\/schema.mathworks.com\\/mf0\\/Connector\\/19700101\"],\"version\":\"1.0\"}"
  power_5_0V1 : Outport  PortName=power_5_0V
  power_12_6V1 : Outport  Port=2  PortName=power_12_6V
  power_21_0V1 : Outport  Port=3  PortName=power_21_0V
  wires:
  Main Battery/1(power_21_0V) -> power_21_0V1/1, BEC/1(power_21_0V)
  BEC/1(power_5_0V) -> power_5_0V1/1
  Payload Battery/1(power_12_6V) -> power_12_6V1/1

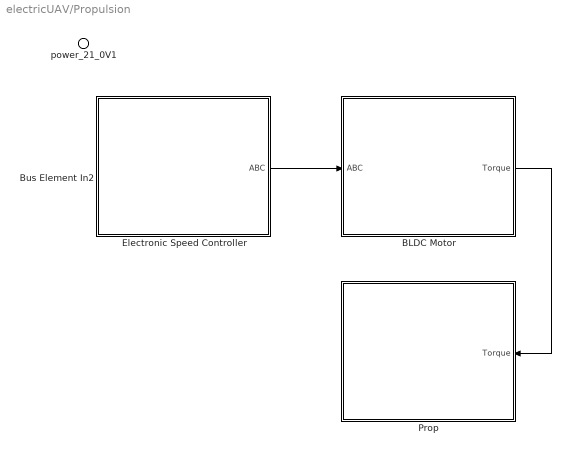
== system electricUAV/Propulsion ==
  power_21_0V1 : Inport  PortName=power_21_0V
  Bus Element In2 : Inport  Port=2  PortName=CtrlCmds  Element=dT
  BLDC Motor : Subsystem
      settings: PortSchema="{\"entries\":[{\"content\":{\"headerSize\":26,\"margin\":15,\"minimumSpacing\":25,\"sides\":[{\"content\":{\"connectorIds\":[\"In1\"]},\"type\":\"ConnectorPlacement.EquallySpacedRectSide\",\"uuid\":\"d39ea880-6caf-4145-b7f0-b92ac95b231c\"},{\"content\":{\"connectorIds\":[\"Out1\"],\"side\":\"RIGHT\"},\"type\":\"ConnectorPlacement.EquallySpacedRectSide\",\"uuid\":\"9a787458-5dfd-4b88-89fa-fa737c2416b2\"},{\"content\":{\"connectorIds\":[],\"side\":\"TOP\"},\"type\":\"ConnectorPlacement.EquallySpacedRectSide\",\"uuid\":\"7005747f-30ee-4956-851b-457a7a1d046d\"}]},\"type\":\"ConnectorPlacement.EquallySpacedConnector\",\"uuid\":\"a95d60af-c1bc-49cc-b537-4a2d2c040baf\"}],\"packageUris\":[\"http:\\/\\/schema.mathworks.com\\/mf0\\/Connector\\/19700101\"],\"version\":\"1.0\"}"
  Electronic Speed Controller : Subsystem
      settings: PortSchema="{\"entries\":[{\"content\":{\"headerSize\":26,\"margin\":15,\"minimumSpacing\":25,\"sides\":[{\"content\":{\"connectorIds\":[]},\"type\":\"ConnectorPlacement.EquallySpacedRectSide\",\"uuid\":\"56b16ad7-3e6c-4ed0-bb60-7867eebb2ed0\"},{\"content\":{\"connectorIds\":[\"Out1\"],\"side\":\"RIGHT\"},\"type\":\"ConnectorPlacement.EquallySpacedRectSide\",\"uuid\":\"9cada59e-5a3c-4135-93c6-afa50d8788cc\"},{\"content\":{\"connectorIds\":[],\"side\":\"TOP\"},\"type\":\"ConnectorPlacement.EquallySpacedRectSide\",\"uuid\":\"af99ad6b-266b-486a-aa1c-385b602e74bb\"}]},\"type\":\"ConnectorPlacement.EquallySpacedConnector\",\"uuid\":\"84df9a0c-2bee-4d18-90ac-1f049874258c\"}],\"packageUris\":[\"http:\\/\\/schema.mathworks.com\\/mf0\\/Connector\\/19700101\"],\"version\":\"1.0\"}"
  Prop : Subsystem
      settings: PortSchema="{\"entries\":[{\"content\":{\"headerSize\":26,\"margin\":15,\"minimumSpacing\":25,\"sides\":[{\"content\":{\"connectorIds\":[]},\"type\":\"ConnectorPlacement.EquallySpacedRectSide\",\"uuid\":\"d39ea880-6caf-4145-b7f0-b92ac95b231c\"},{\"content\":{\"connectorIds\":[\"In1\"],\"side\":\"RIGHT\"},\"type\":\"ConnectorPlacement.EquallySpacedRectSide\",\"uuid\":\"9a787458-5dfd-4b88-89fa-fa737c2416b2\"},{\"content\":{\"connectorIds\":[],\"side\":\"TOP\"},\"type\":\"ConnectorPlacement.EquallySpacedRectSide\",\"uuid\":\"7005747f-30ee-4956-851b-457a7a1d046d\"}]},\"type\":\"ConnectorPlacement.EquallySpacedConnector\",\"uuid\":\"a95d60af-c1bc-49cc-b537-4a2d2c040baf\"}],\"packageUris\":[\"http:\\/\\/schema.mathworks.com\\/mf0\\/Connector\\/19700101\"],\"version\":\"1.0\"}"
  wires:
  BLDC Motor/1(Torque) -> Prop/1(Torque)
  Electronic Speed Controller/1(ABC) -> BLDC Motor/1(ABC)

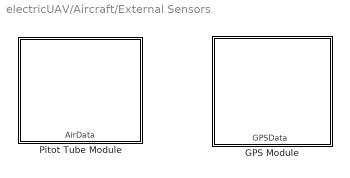
== system electricUAV/Aircraft/External Sensors ==
  GPS Module : Subsystem
      settings: PortSchema="{\"entries\":[{\"content\":{\"headerSize\":26,\"margin\":15,\"minimumSpacing\":25,\"sides\":[{\"content\":{\"connectorIds\":[]},\"type\":\"ConnectorPlacement.EquallySpacedRectSide\",\"uuid\":\"9f35dc00-989c-4612-aee9-27ffd041f5d2\"},{\"content\":{\"connectorIds\":[],\"side\":\"RIGHT\"},\"type\":\"ConnectorPlacement.EquallySpacedRectSide\",\"uuid\":\"fc636a36-c80d-4d26-be49-cb148246bb8f\"},{\"content\":{\"connectorIds\":[],\"side\":\"TOP\"},\"type\":\"ConnectorPlacement.EquallySpacedRectSide\",\"uuid\":\"9fe3dfb0-e690-4d7f-8c9a-5f9d40a5a564\"},{\"content\":{\"connectorIds\":[\"Out1\"],\"side\":\"BOTTOM\"},\"type\":\"ConnectorPlacement.EquallySpacedRectSide\",\"uuid\":\"849be294-e2a5-439f-8ad2-64d927b9f694\"}]},\"type\":\"ConnectorPlacement.EquallySpacedConnector\",\"uuid\":\"46c87048-a43e-442c-ad6b-39b68668708d\"}],\"packageUris\":[\"http:\\/\\/schema.mathworks.com\\/mf0\\/Connector\\/19700101\"],\"version\":\"1.0\"}"
  Pitot Tube Module : Subsystem
      settings: PortSchema="{\"entries\":[{\"content\":{\"headerSize\":26,\"margin\":15,\"minimumSpacing\":25,\"sides\":[{\"content\":{\"connectorIds\":[]},\"type\":\"ConnectorPlacement.EquallySpacedRectSide\",\"uuid\":\"288187f8-f80a-4535-8eff-6998f4e932c0\"},{\"content\":{\"connectorIds\":[],\"side\":\"RIGHT\"},\"type\":\"ConnectorPlacement.EquallySpacedRectSide\",\"uuid\":\"d1e22774-cdd2-4e71-94b1-3e938d9d16f6\"},{\"content\":{\"connectorIds\":[],\"side\":\"TOP\"},\"type\":\"ConnectorPlacement.EquallySpacedRectSide\",\"uuid\":\"890411bd-a9cd-40b1-a683-0574f0cd14d7\"},{\"content\":{\"connectorIds\":[\"Out1\"],\"side\":\"BOTTOM\"},\"type\":\"ConnectorPlacement.EquallySpacedRectSide\",\"uuid\":\"13559410-32ac-48b6-8b1d-f616ead46f43\"}]},\"type\":\"ConnectorPlacement.EquallySpacedConnector\",\"uuid\":\"f677e6f7-ddb0-43ad-ab3a-7892dac74d79\"}],\"packageUris\":[\"http:\\/\\/schema.mathworks.com\\/mf0\\/Connector\\/19700101\"],\"version\":\"1.0\"}"

== system electricUAV/Aircraft/Main Fuselage ==
  Bus Element In2 : Inport  PortName=dR_dE

== system electricUAV/Aircraft/Wings ==
  Bus Element In2 : Inport  PortName=dA

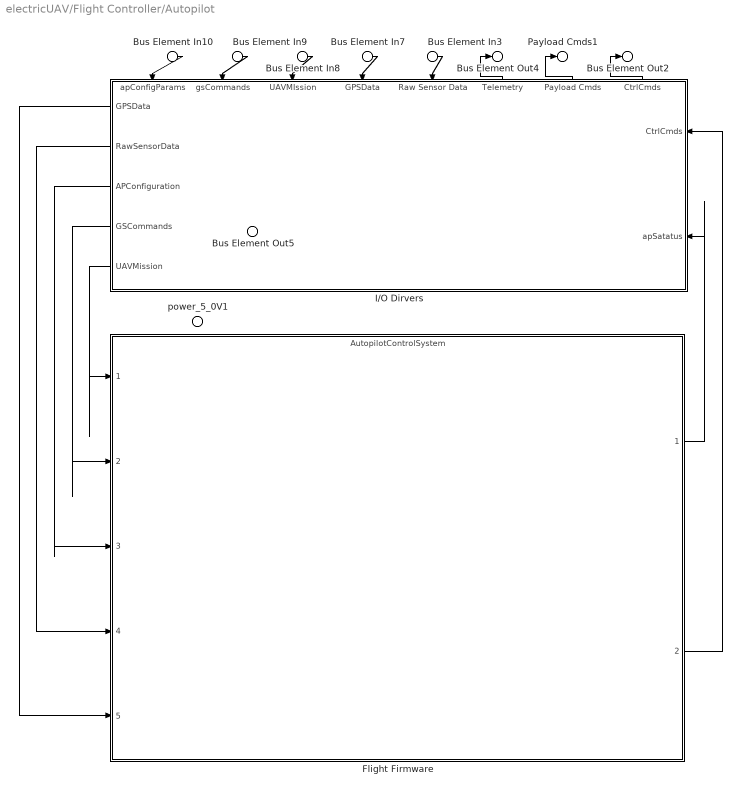
== system electricUAV/Flight Controller/Autopilot ==
  power_5_0V1 : Inport  PortName=power_5_0V
  Bus Element In3 : Inport  Port=2  PortName=Raw Sensor Data
  Bus Element In7 : Inport  Port=3  PortName=GPSData
  Bus Element In8 : Inport  Port=4  PortName=UAVMIssion
  Bus Element In9 : Inport  Port=5  PortName=gsCommands
  Bus Element In10 : Inport  Port=6  PortName=apConfigParams
  Flight Firmware : ModelReference  ModelNameDialog=AutopilotControlSystem  SimulationMode=Normal  ModelReferenceVersion=1.361
      settings: PortSchema="{\"entries\":[{\"content\":{\"headerSize\":38,\"margin\":15,\"minimumSpacing\":25,\"sides\":[{\"content\":{\"connectorIds\":[\"In1\",\"In2\",\"In3\",\"In4\",\"In5\"]},\"type\":\"ConnectorPlacement.EquallySpacedRectSide\",\"uuid\":\"76636d8c-2a71-4cfe-9798-180c72f47694\"},{\"content\":{\"connectorIds\":[\"Out1\",\"Out2\"],\"side\":\"RIGHT\"},\"type\":\"ConnectorPlacement.EquallySpacedRectSide\",\"uuid\":\"872f7c71-0239-4d56-8641-47d463e7d626\"},{\"content\":{\"connectorIds\":[],\"side\":\"TOP\"},\"type\":\"ConnectorPlacement.EquallySpacedRectSide\",\"uuid\":\"1d792a1c-d9fe-46f0-a4cc-898d179764e8\"}]},\"type\":\"ConnectorPlacement.EquallySpacedConnector\",\"uuid\":\"a92a26c6-31c1-4459-9e74-ec0692bdfd16\"}],\"packageUris\":[\"http:\\/\\/schema.mathworks.com\\/mf0\\/Connector\\/19700101\"],\"version\":\"1.0\"}"
  I/O Dirvers : Subsystem
      settings: PortSchema="{\"entries\":[{\"content\":{\"headerSize\":26,\"margin\":15,\"minimumSpacing\":25,\"sides\":[{\"content\":{\"connectorIds\":[\"Out1\",\"Out5\",\"Out6\",\"Out7\",\"Out8\"]},\"type\":\"ConnectorPlacement.EquallySpacedRectSide\",\"uuid\":\"76636d8c-2a71-4cfe-9798-180c72f47694\"},{\"content\":{\"connectorIds\":[\"In2\",\"In1\"],\"side\":\"RIGHT\"},\"type\":\"ConnectorPlacement.EquallySpacedRectSide\",\"uuid\":\"872f7c71-0239-4d56-8641-47d463e7d626\"},{\"content\":{\"connectorIds\":[\"In3\",\"In4\",\"In5\",\"In6\",\"In7\",\"Out4\",\"Out3\",\"Out2\"],\"side\":\"TOP\"},\"type\":\"ConnectorPlacement.EquallySpacedRectSide\",\"uuid\":\"1d792a1c-d9fe-46f0-a4cc-898d179764e8\"},{\"content\":{\"connectorIds\":[],\"side\":\"BOTTOM\"},\"type\":\"ConnectorPlacement.EquallySpacedRectSide\",\"uuid\":\"e2b78097-c2b2-4774-a3d1-9f434413707f\"}]},\"type\":\"ConnectorPlacement.EquallySpacedConnector\",\"uuid\":\"a92a26c6-31c1-4459-9e74-ec0692bdfd16\"}],\"packageUris\":[\"http:\\/\\/schema.mathworks.com\\/mf0\\/Connector\\/19700101\"],\"version\":\"1.0\"}"
  Bus Element Out5 : Outport  PortName=RFSignal
  Bus Element Out2 : Outport  Port=2  PortName=CtrlCmds
  Bus Element Out4 : Outport  Port=3  PortName=Telemetry
  Payload Cmds1 : Outport  Port=4  PortName=Payload Cmds
  wires:
  Bus Element In3/1 -> I/O Dirvers/7(Raw Sensor Data)
  Bus Element In7/1 -> I/O Dirvers/6(GPSData)
  Bus Element In8/1 -> I/O Dirvers/5(UAVMIssion)
  Bus Element In9/1 -> I/O Dirvers/4(gsCommands)
  Bus Element In10/1 -> I/O Dirvers/3(apConfigParams)
  I/O Dirvers/8(UAVMission) -> Flight Firmware/1
  I/O Dirvers/7(GSCommands) -> Flight Firmware/2
  I/O Dirvers/6(APConfiguration) -> Flight Firmware/3
  I/O Dirvers/5(RawSensorData) -> Flight Firmware/4
  I/O Dirvers/1("GPSData ") -> Flight Firmware/5
  Flight Firmware/1 -> I/O Dirvers/1(apSatatus)
  Flight Firmware/2 -> I/O Dirvers/2(CtrlCmds)
  I/O Dirvers/4(Telemetry) -> Bus Element Out4/1
  I/O Dirvers/3(Payload Cmds) -> Payload Cmds1/1
  I/O Dirvers/2("CtrlCmds ") -> Bus Element Out2/1

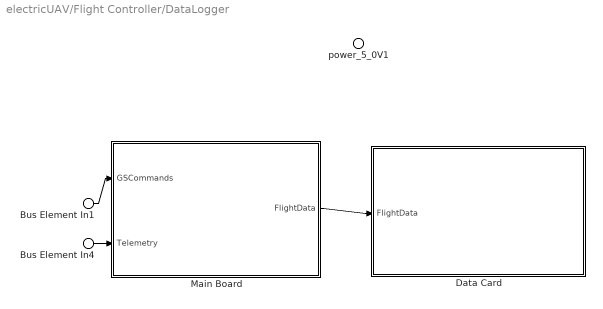
== system electricUAV/Flight Controller/DataLogger ==
  power_5_0V1 : Inport  PortName=power_5_0V
  Bus Element In1 : Inport  Port=2  PortName=GSComms
  Bus Element In4 : Inport  Port=3  PortName=Telemetry
  Data Card : Subsystem
      settings: PortSchema="{\"entries\":[{\"content\":{\"headerSize\":26,\"margin\":15,\"minimumSpacing\":25,\"sides\":[{\"content\":{\"connectorIds\":[\"In1\"]},\"type\":\"ConnectorPlacement.EquallySpacedRectSide\",\"uuid\":\"410c5b0f-08b5-48c1-aeab-ad32707f18cb\"},{\"content\":{\"connectorIds\":[],\"side\":\"RIGHT\"},\"type\":\"ConnectorPlacement.EquallySpacedRectSide\",\"uuid\":\"175f376c-06cb-43d8-93cf-cfe74288c6ca\"},{\"content\":{\"connectorIds\":[],\"side\":\"TOP\"},\"type\":\"ConnectorPlacement.EquallySpacedRectSide\",\"uuid\":\"49daa1ce-2b00-43ab-833d-e4aa679275fe\"}]},\"type\":\"ConnectorPlacement.EquallySpacedConnector\",\"uuid\":\"5fe6ec80-a25e-4dcf-8012-d525fb653d3d\"}],\"packageUris\":[\"http:\\/\\/schema.mathworks.com\\/mf0\\/Connector\\/19700101\"],\"version\":\"1.0\"}"
  Main Board : Subsystem
      settings: PortSchema="{\"entries\":[{\"content\":{\"headerSize\":26,\"margin\":15,\"minimumSpacing\":25,\"sides\":[{\"content\":{\"connectorIds\":[\"In1\",\"In2\"]},\"type\":\"ConnectorPlacement.EquallySpacedRectSide\",\"uuid\":\"410c5b0f-08b5-48c1-aeab-ad32707f18cb\"},{\"content\":{\"connectorIds\":[\"Out1\"],\"side\":\"RIGHT\"},\"type\":\"ConnectorPlacement.EquallySpacedRectSide\",\"uuid\":\"175f376c-06cb-43d8-93cf-cfe74288c6ca\"},{\"content\":{\"connectorIds\":[],\"side\":\"TOP\"},\"type\":\"ConnectorPlacement.EquallySpacedRectSide\",\"uuid\":\"49daa1ce-2b00-43ab-833d-e4aa679275fe\"}]},\"type\":\"ConnectorPlacement.EquallySpacedConnector\",\"uuid\":\"5fe6ec80-a25e-4dcf-8012-d525fb653d3d\"}],\"packageUris\":[\"http:\\/\\/schema.mathworks.com\\/mf0\\/Connector\\/19700101\"],\"version\":\"1.0\"}"
  wires:
  Bus Element In4/1 -> Main Board/2(Telemetry)
  Main Board/1(FlightData) -> Data Card/1(FlightData)
  Bus Element In1/1 -> Main Board/1(GSCommands)

== system electricUAV/Flight Controller/Enclosure ==

== system electricUAV/Flight Controller/Telemetry Antenna ==
  Bus Element In1 : Inport  PortName=RFSignal

== system electricUAV/Payload/Gimbaled Payload ==
  Bus Element In2 : Inport  PortName=operatorCmds  Element=PTZCmds
  Bus Element Out1 : Outport  PortName=Video Out

== system electricUAV/Payload/Payload Data Link ==
  Bus Element In1 : Inport  PortName=Video In
  Bus Element Out1 : Outport  PortName=Data Link

== system electricUAV/Power/BEC ==
  Bus Element In1 : Inport  PortName=power_21_0V
  Bus Element Out1 : Outport  PortName=power_5_0V

== system electricUAV/Power/Main Battery ==
  Bus Element Out1 : Outport  PortName=power_21_0V

== system electricUAV/Power/Payload Battery ==
  Bus Element Out1 : Outport  PortName=power_12_6V

== system electricUAV/Propulsion/BLDC Motor ==
  Bus Element In1 : Inport  PortName=ABC
  Bus Element Out1 : Outport  PortName=Torque

== system electricUAV/Propulsion/Electronic Speed Controller ==
  ABC1 : Outport  PortName=ABC

== system electricUAV/Propulsion/Prop ==
  Bus Element In1 : Inport  PortName=Torque

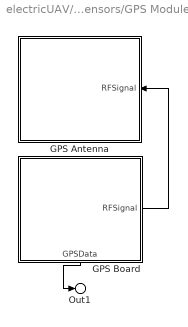
== system electricUAV/Aircraft/External Sensors/GPS Module ==
  GPS Antenna : Subsystem
      settings: PortSchema="{\"entries\":[{\"content\":{\"headerSize\":26,\"margin\":15,\"minimumSpacing\":25,\"sides\":[{\"content\":{\"connectorIds\":[]},\"type\":\"ConnectorPlacement.EquallySpacedRectSide\",\"uuid\":\"1d3f3a23-636b-441d-85a6-b75e05b18389\"},{\"content\":{\"connectorIds\":[\"In1\"],\"side\":\"RIGHT\"},\"type\":\"ConnectorPlacement.EquallySpacedRectSide\",\"uuid\":\"e22d7e46-f58c-4c9d-8892-998381cd60e3\"},{\"content\":{\"connectorIds\":[],\"side\":\"TOP\"},\"type\":\"ConnectorPlacement.EquallySpacedRectSide\",\"uuid\":\"8b16ddbb-b471-4974-8372-55ce1efe9f0b\"}]},\"type\":\"ConnectorPlacement.EquallySpacedConnector\",\"uuid\":\"3aaecc83-0a24-4c0b-b096-52d61c24d002\"}],\"packageUris\":[\"http:\\/\\/schema.mathworks.com\\/mf0\\/Connector\\/19700101\"],\"version\":\"1.0\"}"
  GPS Board : Subsystem
      settings: PortSchema="{\"entries\":[{\"content\":{\"headerSize\":26,\"margin\":15,\"minimumSpacing\":25,\"sides\":[{\"content\":{\"connectorIds\":[]},\"type\":\"ConnectorPlacement.EquallySpacedRectSide\",\"uuid\":\"288187f8-f80a-4535-8eff-6998f4e932c0\"},{\"content\":{\"connectorIds\":[\"Out1\"],\"side\":\"RIGHT\"},\"type\":\"ConnectorPlacement.EquallySpacedRectSide\",\"uuid\":\"d1e22774-cdd2-4e71-94b1-3e938d9d16f6\"},{\"content\":{\"connectorIds\":[],\"side\":\"TOP\"},\"type\":\"ConnectorPlacement.EquallySpacedRectSide\",\"uuid\":\"890411bd-a9cd-40b1-a683-0574f0cd14d7\"},{\"content\":{\"connectorIds\":[\"Out2\"],\"side\":\"BOTTOM\"},\"type\":\"ConnectorPlacement.EquallySpacedRectSide\",\"uuid\":\"27348620-2e46-434a-9ea6-67f85aeb7bd2\"}]},\"type\":\"ConnectorPlacement.EquallySpacedConnector\",\"uuid\":\"f677e6f7-ddb0-43ad-ab3a-7892dac74d79\"}],\"packageUris\":[\"http:\\/\\/schema.mathworks.com\\/mf0\\/Connector\\/19700101\"],\"version\":\"1.0\"}"
  Out1 : Outport  PortName=GPSData
  wires:
  GPS Board/2(GPSData) -> Out1/1
  GPS Board/1(RFSignal) -> GPS Antenna/1(RFSignal)

== system electricUAV/Aircraft/External Sensors/Pitot Tube Module ==
  Bus Element Out1 : Outport  PortName=AirData

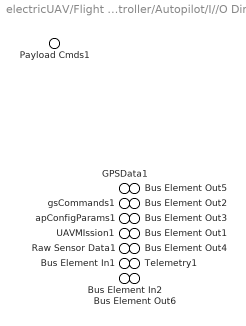
== system electricUAV/Flight Controller/Autopilot/I//O Dirvers ==
  Bus Element In1 : Inport  PortName=apSatatus
  Bus Element In2 : Inport  Port=2  PortName=CtrlCmds
  apConfigParams1 : Inport  Port=3  PortName=apConfigParams
  gsCommands1 : Inport  Port=4  PortName=gsCommands
  UAVMIssion1 : Inport  Port=5  PortName=UAVMIssion
  GPSData1 : Inport  Port=6  PortName=GPSData
  Raw Sensor Data1 : Inport  Port=7  PortName=Raw Sensor Data
  Bus Element Out5 : Outport  PortName=GPSData
  Bus Element Out6 : Outport  Port=2  PortName=CtrlCmds
  Payload Cmds1 : Outport  Port=3  PortName=Payload Cmds
  Telemetry1 : Outport  Port=4  PortName=Telemetry
  Bus Element Out4 : Outport  Port=5  PortName=RawSensorData
  Bus Element Out3 : Outport  Port=6  PortName=APConfiguration
  Bus Element Out2 : Outport  Port=7  PortName=GSCommands
  Bus Element Out1 : Outport  Port=8  PortName=UAVMission
  wires:
  GPSData1/1 -> Bus Element Out5/1
  gsCommands1/1 -> Bus Element Out2/1
  apConfigParams1/1 -> Bus Element Out3/1
  UAVMIssion1/1 -> Bus Element Out1/1
  Raw Sensor Data1/1 -> Bus Element Out4/1
  Bus Element In1/1 -> Telemetry1/1
  Bus Element In2/1 -> Bus Element Out6/1

== system electricUAV/Flight Controller/DataLogger/Data Card ==
  Bus Element In1 : Inport  PortName=FlightData

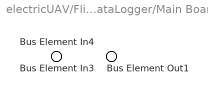
== system electricUAV/Flight Controller/DataLogger/Main Board ==
  Bus Element In3 : Inport  PortName=GSCommands
  Bus Element In4 : Inport  Port=2  PortName=Telemetry
  Bus Element Out1 : Outport  PortName=FlightData

== system electricUAV/Aircraft/External Sensors/GPS Module/GPS Antenna ==
  Bus Element In1 : Inport  PortName=RFSignal

== system electricUAV/Aircraft/External Sensors/GPS Module/GPS Board ==
  Bus Element Out2 : Outport  PortName=RFSignal
  Bus Element Out1 : Outport  Port=2  PortName=GPSData
